simulink model "drone_easy_v2"  (R2021a)
settings: Solver=VariableStepAuto  StartTime=0.0  StopTime=1  RelTol=1e-3
undefined symbols (not defined in the file or in its folder): params
settings Model: Creator=FusionLab  LastModifiedBy=FusionLab

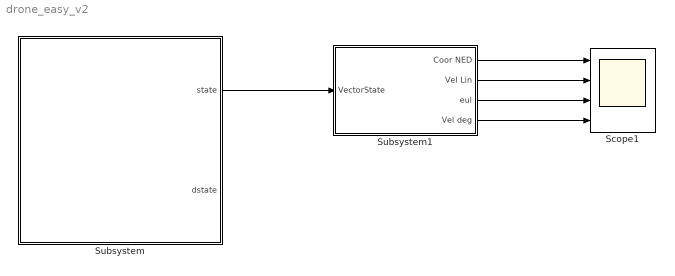
== system drone_easy_v2 ==
  Scope1 : Scope  NumInputPorts=4
  Subsystem : Subsystem
  Subsystem1 : Subsystem
  wires:
  Subsystem1/4(Vel deg) -> Scope1/4
  Subsystem1/3(eul) -> Scope1/3
  Subsystem1/2(Vel Lin) -> Scope1/2
  Subsystem1/1(Coor NED) -> Scope1/1
  Subsystem/1(state) -> Subsystem1/1(VectorState)

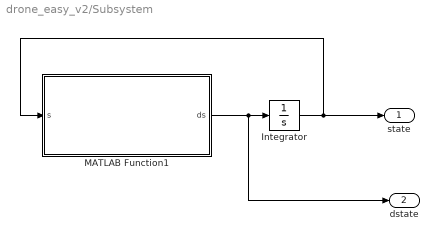
== system drone_easy_v2/Subsystem ==
  Integrator : Integrator  InitialCondition=params.s0
  MATLAB Function1 : MATLAB Function  TreatAsAtomicUnit=on
  state : Outport
  dstate : Outport  Port=2
  wires:
  MATLAB Function1/1(ds) -> dstate/1, Integrator/1
  Integrator/1 -> state/1, MATLAB Function1/1(s)

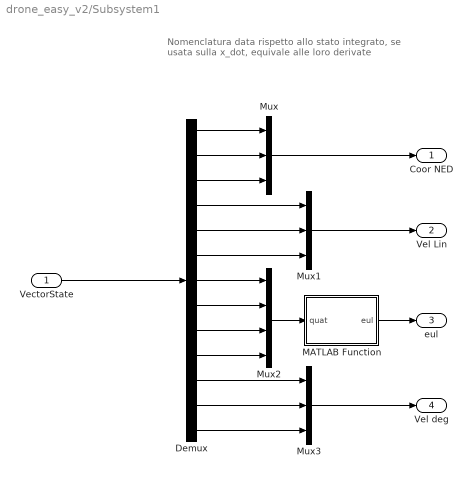
== system drone_easy_v2/Subsystem1 ==
  note: Nomenclatura data rispetto allo stato integrato, se usata sulla x_dot, equivale alle loro derivate
  VectorState : Inport
  Demux : Demux  Outputs=13
  MATLAB Function : MATLAB Function  TreatAsAtomicUnit=on
  Mux : Mux  Inputs=3
  Mux1 : Mux  Inputs=3
  Mux2 : Mux
  Mux3 : Mux  Inputs=3
  Coor NED : Outport
  Vel Lin : Outport  Port=2
  eul : Outport  Port=3
  Vel deg : Outport  Port=4
  wires:
  Demux/11 -> Mux3/1
  Demux/8 -> Mux2/2
  Mux/1 -> Coor NED/1
  Demux/6 -> Mux1/3
  Demux/9 -> Mux2/3
  Demux/1 -> Mux/1
  Demux/12 -> Mux3/2
  Demux/10 -> Mux2/4
  Demux/4 -> Mux1/1
  Demux/13 -> Mux3/3
  Demux/5 -> Mux1/2
  VectorState/1 -> Demux/1
  Demux/2 -> Mux/2
  Demux/7 -> Mux2/1
  Demux/3 -> Mux/3
  Mux1/1 -> Vel Lin/1
  Mux3/1 -> Vel deg/1
  MATLAB Function/1(eul) -> eul/1
  Mux2/1 -> MATLAB Function/1(quat)

== matlab function drone_easy_v2/Subsystem1/MATLAB Function ==
  data: quat input; eul output
function eul = quat2eul(quat)
a = quat2eul(quat');
eul=a';
end

== matlab function drone_easy_v2/Subsystem/MATLAB Function1 ==
  data: ds output; s input; params parameter
function ds = Dynamics_v1(s, params)



% Initialize integration vectors and parameters

ds = zeros(size(s));

%s= [x y z q0 q1 q2 q3 u v w p q r]

% Extract attitude, angular velocity 
q =  s(4:7);
omega= s(11:13);

%position, linear velocity
ned=s(1:3);
vel=s(8:10);

%quat2eul
eul=quat2eul(q');


%%%%%%%%%%%%%%%%%% Attitude Kinematics Equations (Quaternions) %%%%%%%%%%%%%%%%%%
Om = [0, -omega(1), -omega(2), -omega(3);
    omega(1), 0, omega(3), -omega(2);
    omega(2), -omega(3), 0, omega(1);
    omega(3), omega(2), -omega(1), 0];

ds(4:7,1) = 0.5*Om*q;

omega_thrust = 0.159155*params.omegaThrust;

Mx=params.l*params.b*(omega_thrust(2)^2-omega_thrust(4)^2);
My=params.l*params.b*(omega_thrust(1)^2-omega_thrust(3)^2);
Mz=params.d*(omega_thrust(1)^2-omega_thrust(2)^2+omega_thrust(3)^2-omega_thrust(4)^2);


pdot=(Mx/params.I(1,1))-omega(2)*omega(3)*(params.I(3,3)-params.I(2,2))/params.I(1,1);
qdot=(My/params.I(1,1))-omega(1)*omega(3)*(params.I(1,1)-params.I(3,3))/params.I(2,2);
rdot=(Mz/params.I(3,3));
ds(11:13)=[pdot; qdot; rdot];


%%%%%%%%%%%%%%Position Kinematics Equation (Eulero)%%%%%%%%%%%
R_out=R(eul);
ds(1:3)=R_out*vel; %xdot ydot zdot

omega_thrust = 0.159155*params.omegaThrust;
T = (params.b*(omega_thrust(1)^2 + omega_thrust(2)^2 + omega_thrust(3)^2 + omega_thrust(4)^2));


 udot=omega(3)*vel(2)-omega(2)*vel(3)-params.g*sin(eul(2));
 vdot=omega(1)*vel(3)-omega(3)*vel(1)-params.g*cos(eul(2))*sin(eul(1));
 wdot=omega(2)*vel(1)-omega(1)*vel(2)+params.g*cos(eul(1))*cos(eul(2))-T/params.m;


ds(8:10)=[udot;vdot;wdot];

end
